simulink model "questao3"  (R2021b)
settings: Solver=VariableStepAuto  StartTime=0.0  StopTime=1800  RelTol=1e-3
values from neighbouring files (symbols this model uses):
  dF = 0    [main.m]
  dFj = 4.72e-5    (= 4.72e-05)    [main.m]
  dTi = 0    [main.m]
  dTij = 0    [main.m]
  G = p*Bu    [main.m]
  Gd1 = p*[Bd11 ... (first row only)    [main.m]
  Gd2 = p*[Bd12 ... (first row only)    [main.m]
  Gd3 = p*[Bd13 ... (first row only)    [main.m]
  Ts = 51.67    [main.m]
settings Model: Creator=luang  LastModifiedBy=luang

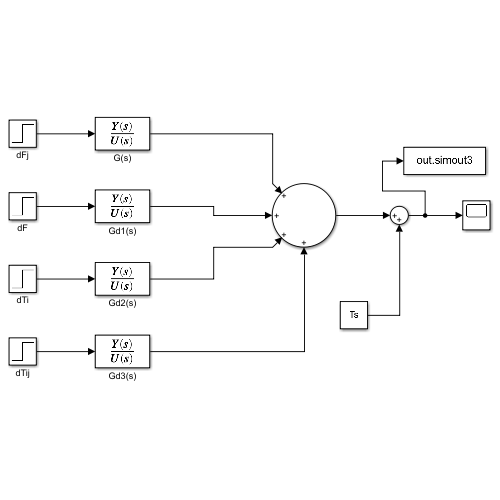
[thumbnail: Simulink's stored preview of the top-level diagram]
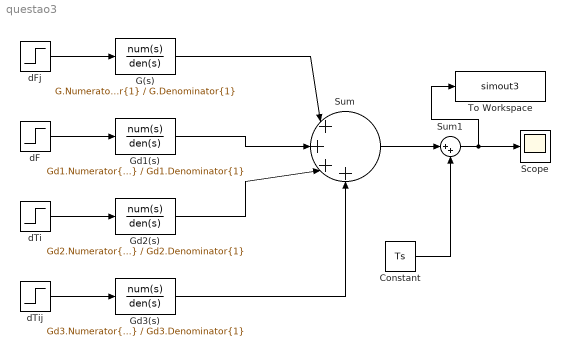
== system questao3 ==
  Constant : Constant  Value=Ts
  G(s) : TransferFcn  Numerator=G.Numerator{1}  Denominator=G.Denominator{1}
  Gd1(s) : TransferFcn  Numerator=Gd1.Numerator{1}  Denominator=Gd1.Denominator{1}
  Gd2(s) : TransferFcn  Numerator=Gd2.Numerator{1}  Denominator=Gd2.Denominator{1}
  Gd3(s) : TransferFcn  Numerator=Gd3.Numerator{1}  Denominator=Gd3.Denominator{1}
  Scope : Scope
  Sum : Sum  Inputs=|++++
  Sum1 : Sum  Inputs=|++
  To Workspace : ToWorkspace  VariableName=simout3  SaveFormat=Structure With Time  SampleTime=-1
  dF : Step  After=dF  SampleTime=0
  dFj : Step  After=dFj  SampleTime=0
  dTi : Step  After=dTi  SampleTime=0
  dTij : Step  After=dTij  SampleTime=0
  wires:
  dFj/1 -> G(s)/1
  dF/1 -> Gd1(s)/1
  dTi/1 -> Gd2(s)/1
  dTij/1 -> Gd3(s)/1
  G(s)/1 -> Sum/1
  Gd1(s)/1 -> Sum/2
  Gd2(s)/1 -> Sum/3
  Gd3(s)/1 -> Sum/4
  Sum/1 -> Sum1/1
  Constant/1 -> Sum1/2
  Sum1/1 -> To Workspace/1, Scope/1
